simulink subsystem "Orientation"  (R2023b)
settings: Solver=VariableStepAuto  StartTime=0.0  StopTime=10.0  RelTol=1e-3
undefined symbols (not defined in the file or in its folder): DiscIntNeverNeededParam, J, w_wheel1, w_wheel2, w_wheel3
libraries: aerolibutil x3, matrix_library x2, sharedtransform x1, dspmtrx3 x1
settings Model: Creator=andrea  LastModifiedBy=andrea

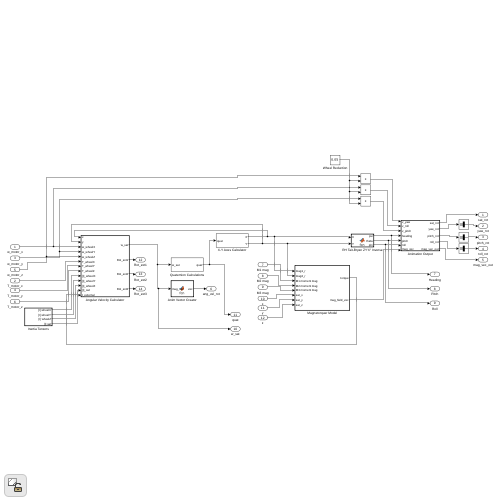
[thumbnail: Simulink's stored preview of the top-level diagram]
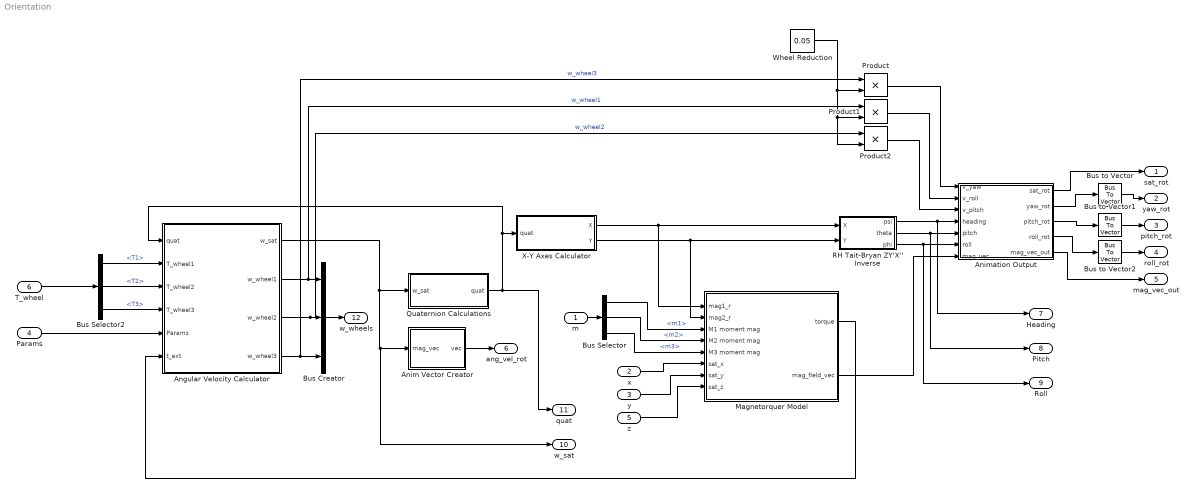
== system Orientation ==
  m : Inport
  x : Inport  Port=2
  y : Inport  Port=3
  Params : Inport  Port=4
  z : Inport  Port=5
  T_wheel : Inport  Port=6
  Angular Velocity Calculator : Subsystem  TreatAsAtomicUnit=on
  Anim Vector Creator : MATLAB Function  TreatAsAtomicUnit=on
  Animation Output : Subsystem  TreatAsAtomicUnit=on
  Bus Creator : BusCreator  Inputs=w_wheel1,w_wheel2,w_wheel3
  Bus Selector : BusSelector  OutputSignals=m1,m2,m3
  Bus Selector2 : BusSelector  OutputSignals=T1,T2,T3
  Bus to Vector : BusToVector
  Bus to Vector1 : BusToVector
  Bus to Vector2 : BusToVector
  Magnetorquer Model : Subsystem  TreatAsAtomicUnit=on
  Product : Product
  Product1 : Product
  Product2 : Product
  Quaternion Calculations : Subsystem
  RH Tait-Bryan ZY'X'' Inverse : MATLAB Function  TreatAsAtomicUnit=on
  Wheel Reduction : Constant  Value=0.05
  X-Y Axes Calculator : Subsystem
  sat_rot : Outport
  yaw_rot : Outport  Port=2
  pitch_rot : Outport  Port=3
  roll_rot : Outport  Port=4
  mag_vec_out : Outport  Port=5
  ang_vel_rot : Outport  Port=6
  Heading : Outport  Port=7
  Pitch : Outport  Port=8
  Roll : Outport  Port=9
  w_sat : Outport  Port=10
  quat : Outport  Port=11
  w_wheels : Outport  Port=12
  wires:
  Animation Output/4(roll_rot) -> Bus to Vector2/1
  Animation Output/3(pitch_rot) -> Bus to Vector1/1
  Bus to Vector1/1 -> pitch_rot/1
  x/1 -> Magnetorquer Model/6(sat_x)
  RH Tait-Bryan ZY'X'' Inverse/3(phi) -> Roll/1, Animation Output/6(roll)
  Wheel Reduction/1 -> Product/2, Product1/2, Product2/2
  Animation Output/1(sat_rot) -> sat_rot/1
  Product1/1 -> Animation Output/2(v_roll)
  Quaternion Calculations/1(quat) -> quat/1, X-Y Axes Calculator/1(quat), Angular Velocity Calculator/1(quat)
  Bus Selector/2 -> Magnetorquer Model/4(M2 moment mag)  "<m2>"
  Angular Velocity Calculator/1(w_sat) -> Anim Vector Creator/1(mag_vec), w_sat/1, Quaternion Calculations/1(w_sat)
  y/1 -> Magnetorquer Model/7(sat_y)
  X-Y Axes Calculator/1(X) -> Magnetorquer Model/1(mag1_r), RH Tait-Bryan ZY'X'' Inverse/1(X)
  z/1 -> Magnetorquer Model/8(sat_z)
  Bus Selector/3 -> Magnetorquer Model/5(M3 moment mag)  "<m3>"
  Bus Selector2/1 -> Angular Velocity Calculator/2(T_wheel1)  "<T1>"
  RH Tait-Bryan ZY'X'' Inverse/2(theta) -> Animation Output/5(pitch), Pitch/1
  Animation Output/5(mag_vec_out) -> mag_vec_out/1
  Bus to Vector2/1 -> roll_rot/1
  Product/1 -> Animation Output/1(v_yaw)
  Animation Output/2(yaw_rot) -> Bus to Vector/1
  Anim Vector Creator/1(vec) -> ang_vel_rot/1
  Product2/1 -> Animation Output/3(v_pitch)
  Bus Selector/1 -> Magnetorquer Model/3(M1 moment mag)  "<m1>"
  RH Tait-Bryan ZY'X'' Inverse/1(psi) -> Heading/1, Animation Output/4(heading)
  X-Y Axes Calculator/2(Y) -> Magnetorquer Model/2(mag2_r), RH Tait-Bryan ZY'X'' Inverse/2(Y)
  Bus to Vector/1 -> yaw_rot/1
  Magnetorquer Model/2(mag_field_vec) -> Animation Output/7(mag_vec)
  Angular Velocity Calculator/2(w_wheel1) -> Bus Creator/1, Product1/1  "w_wheel1"
  Angular Velocity Calculator/3(w_wheel2) -> Bus Creator/2, Product2/1  "w_wheel2"
  Angular Velocity Calculator/4(w_wheel3) -> Bus Creator/3, Product/1  "w_wheel3"
  m/1 -> Bus Selector/1
  T_wheel/1 -> Bus Selector2/1
  Bus Creator/1 -> w_wheels/1
  Params/1 -> Angular Velocity Calculator/5(Params)
  Bus Selector2/2 -> Angular Velocity Calculator/3(T_wheel2)  "<T2>"
  Bus Selector2/3 -> Angular Velocity Calculator/4(T_wheel3)  "<T3>"
  Magnetorquer Model/1(torque) -> Angular Velocity Calculator/6(t_ext)

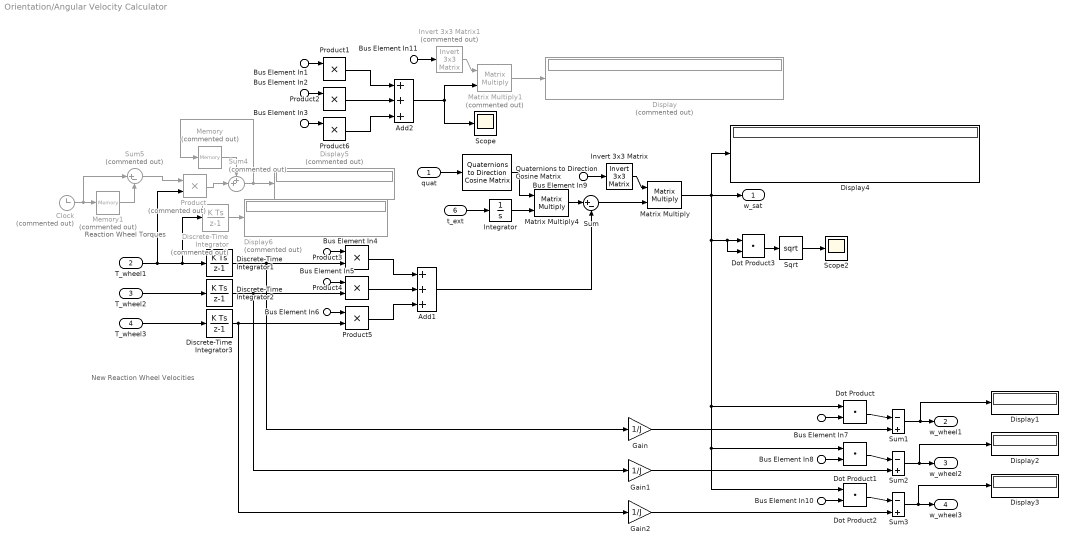
== system Orientation/Angular Velocity Calculator ==
  note: New Reaction Wheel Velocities
  note: Reaction Wheel Torques
  quat : Inport
  T_wheel1 : Inport  Port=2
  T_wheel2 : Inport  Port=3
  T_wheel3 : Inport  Port=4
  Bus Element In9 : Inport  Port=5  PortName=Params  Element=I_sat
  Bus Element In11 : Inport  Port=5  PortName=Params  Element=I_sat
  Bus Element In4 : Inport  Port=5  PortName=Params  Element=a1
  Bus Element In7 : Inport  Port=5  PortName=Params  Element=a1
  Bus Element In1 : Inport  Port=5  PortName=Params  Element=a1
  Bus Element In5 : Inport  Port=5  PortName=Params  Element=a2
  Bus Element In8 : Inport  Port=5  PortName=Params  Element=a2
  Bus Element In2 : Inport  Port=5  PortName=Params  Element=a2
  Bus Element In6 : Inport  Port=5  PortName=Params  Element=a3
  Bus Element In10 : Inport  Port=5  PortName=Params  Element=a3
  Bus Element In3 : Inport  Port=5  PortName=Params  Element=a3
  t_ext : Inport  Port=6
  Add1 : Sum  Inputs=+++
  Add2 : Sum  Inputs=+++
  Clock : Clock  Commented=on
  Discrete-Time Integrator : DiscreteIntegrator  Commented=on  SampleTime=-1  ICPrevOutput=DiscIntNeverNeededParam  ICPrevScaledInput=DiscIntNeverNeededParam
  Discrete-Time Integrator1 : DiscreteIntegrator  SampleTime=-1  ICPrevOutput=DiscIntNeverNeededParam  ICPrevScaledInput=DiscIntNeverNeededParam
  Discrete-Time Integrator2 : DiscreteIntegrator  SampleTime=-1  ICPrevOutput=DiscIntNeverNeededParam  ICPrevScaledInput=DiscIntNeverNeededParam
  Discrete-Time Integrator3 : DiscreteIntegrator  SampleTime=-1  ICPrevOutput=DiscIntNeverNeededParam  ICPrevScaledInput=DiscIntNeverNeededParam
  Display : Display  Commented=on
  Display{1..4} (4 alike) : Display
  Display5 : Display  Commented=on
  Display6 : Display  Commented=on
  Dot Product{,1..3} (4 alike) : DotProduct  OutDataTypeStr=Inherit: Inherit via internal rule
  Gain : Gain  Gain=1/J
  Gain1 : Gain  Gain=1/J
  Gain2 : Gain  Gain=1/J
  Integrator : Integrator
  Invert 3x3 Matrix : aerolibutil/Invert  3x3 Matrix
  Invert 3x3 Matrix1 : aerolibutil/Invert  3x3 Matrix  Commented=on
  Matrix Multiply : Product  Multiplication=Matrix(*)
  Matrix Multiply1 : Product  Commented=on  Multiplication=Matrix(*)
  Matrix Multiply4 : Product  Multiplication=Matrix(*)
  Memory : Memory  Commented=on
  Memory1 : Memory  Commented=on
  Product : Product  Commented=on
  Product{1..6} (6 alike) : Product
  Quaternions to Direction Cosine Matrix : sharedtransform/Quaternions to  Direction Cosine Matrix  aMode=aMode
      settings: LibrarySourceBlock=|
      | aerolibtransform2/Quaternions to
      | Direction Cosine Matrix
  Scope : Scope
  Scope2 : Scope
  Sqrt : Sqrt
  Sum : Sum  Inputs=|+-
  Sum1 : Sum  Inputs=-|+
  Sum2 : Sum  Inputs=-|+
  Sum3 : Sum  Inputs=-|+
  Sum4 : Sum  Commented=on  Inputs=++|
  Sum5 : Sum  Commented=on  Inputs=|+-
  w_sat : Outport
  w_wheel1 : Outport  Port=2
  w_wheel2 : Outport  Port=3
  w_wheel3 : Outport  Port=4
  wires:
  Discrete-Time Integrator/1 -> Display6/1
  T_wheel1/1 -> Discrete-Time Integrator/1, Discrete-Time Integrator1/1, Product/2
  Product/1 -> Sum4/2
  Sum5/1 -> Product/1
  Memory1/1 -> Sum5/2
  Clock/1 -> Memory1/1, Sum5/1
  Sum4/1 -> Memory/1, Display5/1
  Memory/1 -> Sum4/1
  Sqrt/1 -> Scope2/1
  Dot Product3/1 -> Sqrt/1
  Matrix Multiply1/1 -> Display/1
  Add2/1 -> Matrix Multiply1/2, Scope/1
  Bus Element In11/1 -> Invert 3x3 Matrix1/1
  Invert 3x3 Matrix1/1 -> Matrix Multiply1/1
  Bus Element In3/1 -> Product6/1
  Product2/1 -> Add2/2
  Bus Element In2/1 -> Product2/1
  Product6/1 -> Add2/3
  Bus Element In1/1 -> Product1/1
  Product1/1 -> Add2/1
  Matrix Multiply/1 -> Dot Product3/1, Dot Product3/2, Dot Product1/1, Dot Product2/1, Dot Product/1, w_sat/1, Display4/1
  Discrete-Time Integrator3/1 -> Product5/2, Gain2/1
  Discrete-Time Integrator2/1 -> Product4/2, Gain1/1
  Discrete-Time Integrator1/1 -> Product3/2, Gain/1
  Invert 3x3 Matrix/1 -> Matrix Multiply/1
  Sum/1 -> Matrix Multiply/2
  Bus Element In9/1 -> Invert 3x3 Matrix/1
  Matrix Multiply4/1 -> Sum/1
  Integrator/1 -> Matrix Multiply4/2
  Quaternions to Direction Cosine Matrix/1 -> Matrix Multiply4/1
  Add1/1 -> Sum/2
  Gain2/1 -> Sum3/2
  Gain1/1 -> Sum2/2
  Gain/1 -> Sum1/2
  T_wheel3/1 -> Discrete-Time Integrator3/1
  T_wheel2/1 -> Discrete-Time Integrator2/1
  t_ext/1 -> Integrator/1
  quat/1 -> Quaternions to Direction Cosine Matrix/1
  Sum3/1 -> Display3/1, w_wheel3/1
  Sum2/1 -> w_wheel2/1, Display2/1
  Sum1/1 -> w_wheel1/1, Display1/1
  Dot Product2/1 -> Sum3/1
  Dot Product1/1 -> Sum2/1
  Dot Product/1 -> Sum1/1
  Bus Element In10/1 -> Dot Product2/2
  Bus Element In8/1 -> Dot Product1/2
  Bus Element In7/1 -> Dot Product/2
  Bus Element In4/1 -> Product3/1
  Bus Element In5/1 -> Product4/1
  Bus Element In6/1 -> Product5/1
  Product5/1 -> Add1/3
  Product3/1 -> Add1/1
  Product4/1 -> Add1/2

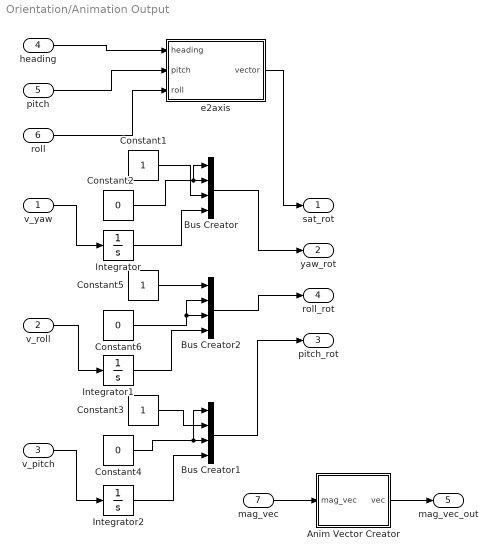
== system Orientation/Animation Output ==
  v_yaw : Inport
  v_roll : Inport  Port=2
  v_pitch : Inport  Port=3
  heading : Inport  Port=4
  pitch : Inport  Port=5
  roll : Inport  Port=6
  mag_vec : Inport  Port=7
  Anim Vector Creator : MATLAB Function  TreatAsAtomicUnit=on
  Bus Creator : BusCreator  Inputs=4
  Bus Creator1 : BusCreator  Inputs=4
  Bus Creator2 : BusCreator  Inputs=4
  Constant1 : Constant
  Constant2 : Constant  Value=0
  Constant3 : Constant
  Constant4 : Constant  Value=0
  Constant5 : Constant
  Constant6 : Constant  Value=0
  Integrator : Integrator
  Integrator1 : Integrator
  Integrator2 : Integrator
  e2axis : MATLAB Function  TreatAsAtomicUnit=on
  sat_rot : Outport
  yaw_rot : Outport  Port=2
  pitch_rot : Outport  Port=3
  roll_rot : Outport  Port=4
  mag_vec_out : Outport  Port=5
  wires:
  Anim Vector Creator/1(vec) -> mag_vec_out/1
  mag_vec/1 -> Anim Vector Creator/1(mag_vec)
  Integrator2/1 -> Bus Creator1/4
  Integrator1/1 -> Bus Creator2/4
  Integrator/1 -> Bus Creator/4
  Bus Creator1/1 -> pitch_rot/1
  Bus Creator2/1 -> roll_rot/1
  Bus Creator/1 -> yaw_rot/1
  v_pitch/1 -> Integrator2/1
  v_roll/1 -> Integrator1/1
  v_yaw/1 -> Integrator/1
  e2axis/1(vector) -> sat_rot/1
  roll/1 -> e2axis/3(roll)
  pitch/1 -> e2axis/2(pitch)
  heading/1 -> e2axis/1(heading)
  Constant4/1 -> Bus Creator1/3, Bus Creator1/1
  Constant2/1 -> Bus Creator/2, Bus Creator/1
  Constant3/1 -> Bus Creator1/2
  Constant1/1 -> Bus Creator/3
  Constant5/1 -> Bus Creator2/1
  Constant6/1 -> Bus Creator2/3, Bus Creator2/2

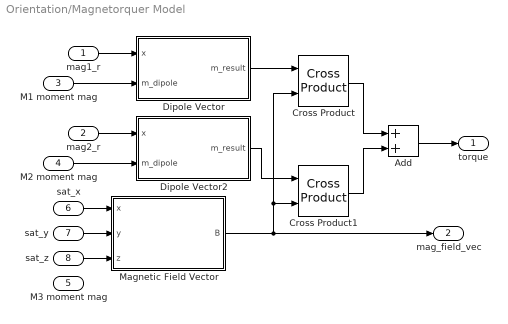
== system Orientation/Magnetorquer Model ==
  mag1_r : Inport
  mag2_r : Inport  Port=2
  M1 moment mag : Inport  Port=3
  M2 moment mag : Inport  Port=4
  M3 moment mag : Inport  Port=5
  sat_x : Inport  Port=6
  sat_y : Inport  Port=7
  sat_z : Inport  Port=8
  Add : Sum
  Cross Product : matrix_library/Cross Product
  Cross Product1 : matrix_library/Cross Product
  Dipole Vector : MATLAB Function  TreatAsAtomicUnit=on
  Dipole Vector2 : MATLAB Function  TreatAsAtomicUnit=on
  Magnetic Field Vector : MATLAB Function  TreatAsAtomicUnit=on
  torque : Outport
  mag_field_vec : Outport  Port=2
  wires:
  mag1_r/1 -> Dipole Vector/1(x)
  mag2_r/1 -> Dipole Vector2/1(x)
  Add/1 -> torque/1
  Dipole Vector/1(m_result) -> Cross Product/1
  M2 moment mag/1 -> Dipole Vector2/2(m_dipole)
  Magnetic Field Vector/1(B) -> Cross Product1/2, Cross Product/2, mag_field_vec/1
  sat_y/1 -> Magnetic Field Vector/2(y)
  sat_z/1 -> Magnetic Field Vector/3(z)
  sat_x/1 -> Magnetic Field Vector/1(x)
  Dipole Vector2/1(m_result) -> Cross Product1/1
  Cross Product/1 -> Add/1
  M1 moment mag/1 -> Dipole Vector/2(m_dipole)
  Cross Product1/1 -> Add/2

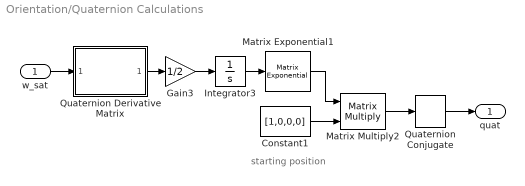
== system Orientation/Quaternion Calculations ==
  note: starting position
  w_sat : Inport
  Constant1 : Constant  Value=[1,0,0,0]
  Gain3 : Gain  Gain=1/2
  Integrator3 : Integrator  InitialCondition=[[0,0,0,0];[0,0,0,0];[0,0,0,0];[0,0,0,0]]
  Matrix Exponential1 : dspmtrx3/Matrix Exponential
  Matrix Multiply2 : Product  Multiplication=Matrix(*)
  Quaternion Conjugate : aerolibutil/Quaternion Conjugate
  Quaternion Derivative Matrix : MATLAB Function  TreatAsAtomicUnit=on
  quat : Outport
  wires:
  Quaternion Conjugate/1 -> quat/1
  w_sat/1 -> Quaternion Derivative Matrix/1(omega)
  Matrix Multiply2/1 -> Quaternion Conjugate/1
  Integrator3/1 -> Matrix Exponential1/1
  Constant1/1 -> Matrix Multiply2/2
  Matrix Exponential1/1 -> Matrix Multiply2/1
  Gain3/1 -> Integrator3/1
  Quaternion Derivative Matrix/1(Omega) -> Gain3/1

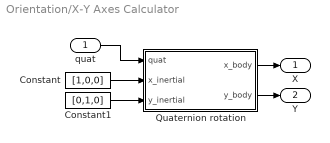
== system Orientation/X-Y Axes Calculator ==
  quat : Inport
  Constant : Constant  Value=[1,0,0]
  Constant1 : Constant  Value=[0,1,0]
  Quaternion rotation : MATLAB Function  TreatAsAtomicUnit=on
  X : Outport
  Y : Outport  Port=2
  wires:
  Quaternion rotation/2(y_body) -> Y/1
  Quaternion rotation/1(x_body) -> X/1
  Constant1/1 -> Quaternion rotation/3(y_inertial)
  Constant/1 -> Quaternion rotation/2(x_inertial)
  quat/1 -> Quaternion rotation/1(quat)

== matlab function Orientation/Animation Output/Anim Vector Creator ==
  data: mag_vec input; vec output
function vec = fcn(mag_vec)

cos_theta = mag_vec(3) / sqrt(mag_vec(1)^2+mag_vec(2)^2+mag_vec(3)^2);
theta = acos(cos_theta);
vec = [-mag_vec(2); mag_vec(1); 0; theta];

== matlab function Orientation/Animation Output/e2axis ==
  data: heading input; pitch input; roll input; vector output

function vector = e2axis(heading, pitch, roll)

eul = [heading -pitch roll];
coder.extrinsic('eul2rotm');
coder.extrinsic('rotm2axang');
rotm = eul2rotm(eul,'ZYX');
v = rotm2axang(rotm);
vector = [0;0;0;0];
vector(1) = v(1);
vector(2) = v(2);
vector(3) = v(3);
vector(4) = v(4);

end

== matlab function Orientation/Magnetorquer Model/Dipole Vector ==
  data: x input; m_result output; m_dipole input
function m_result  = fcn(x,m_dipole)

m_result = [0;0;0];
mag = sqrt(x(1)^2 + x(2)^2 + x(3)^2);
m_result(1) = m_dipole * (x(1) / mag);
m_result(2) = m_dipole * (x(2) / mag);
m_result(3) = m_dipole * (x(3) / mag);

== matlab function Orientation/Magnetorquer Model/Dipole Vector2 ==
  data: x input; m_result output; m_dipole input
function m_result  = fcn(x,m_dipole)

m_result = [0;0;0];
mag = sqrt(x(1)^2 + x(2)^2 + x(3)^2);
m_result(1) = m_dipole * (x(1) / mag);
m_result(2) = m_dipole * (x(2) / mag);
m_result(3) = m_dipole * (x(3) / mag);

== matlab function Orientation/Magnetorquer Model/Magnetic Field Vector ==
  data: x input; B output; y input; z input
function B  = fcn(x,y,z)

B = [0;0;0];
q1 = 150; % bottom charge
q2 = 180; % top charge
r_earth = 6.3781e6;
inset = 2/3;
d_t = x^2 + y^2 + (z - r_earth * inset)^2; % distance squared from top charge to point
d_b = x^2 + y^2 + (z + r_earth * inset)^2; % distance squared from bottom charge to point

B(1) = (x) * (q1 / d_b - q2 / d_t);
B(2) = (y) * (q1 / d_b - q2 / d_t);
B(3) = (q1 / d_b) * (z + r_earth * inset) - (q1 / d_t) * (z - r_earth * inset);

== matlab function Orientation/Quaternion Calculations/Quaternion Derivative Matrix ==
  data: omega input; Omega output
function Omega = fcn(omega)

omega_cell = num2cell(omega);
[omega_x, omega_y, omega_z] = omega_cell{:};

%omega_x = omega(1);
%omega_y = omega(2);
%omega_z = omega(3);

Omega = [[0,            -omega_x,   -omega_y,   -omega_z];
         [omega_x,      0,          -omega_z,    omega_y];
         [omega_y,      omega_z,    0,          -omega_x];
         [omega_z,      -omega_y,   omega_x,    0       ]];

== matlab function Orientation/X-Y Axes Calculator/Quaternion rotation ==
  data: quat input; x_body output; x_inertial input; y_inertial input; y_body output
function [x_body, y_body] = fcn(quat, x_inertial, y_inertial)

x_body = [0,0,0];
y_body = [0,0,0];

%disp("Quaternion:");
%disp(reshape(quat,1,4));
%fprintf(quat);
coder.extrinsic("quat2dcm");
dcm = quat2dcm(reshape(quat,1,4));

x_body = reshape(dcm * x_inertial,1,3);
y_body = reshape(dcm * y_inertial,1,3);


% z_body = x_body x y_body

== matlab function Orientation/Anim Vector Creator ==
  data: mag_vec input; vec output
function vec = fcn(mag_vec)

cos_theta = mag_vec(3) / sqrt(mag_vec(1)^2+mag_vec(2)^2+mag_vec(3)^2);
theta = acos(cos_theta);
vec = [-mag_vec(2); mag_vec(1); 0; theta];

== matlab function Orientation/RH Tait-Bryan ZY'X'' Inverse ==
  data: X input; psi output; theta output; phi output; Y input
function [psi, theta, phi] = fcn(X, Y)

% psi = heading
% theta = pitch
% phi = bank

%eulZYX = [0,0,0];
%coder.extrinsic("quat2eul");
%eulZYX = quat2eul(reshape(quat,1,4));

%psi = eulZYX(1);
%theta = eulZYX(2);
%phi = eulZYX(3);

psi = atan2(X(2),X(1));
theta = atan2(X(3),sqrt(X(2)^2 + X(1)^2));
if(-Y(1) * sin(psi) + Y(2) * cos(psi) > 1)
    n = 1;
elseif(-Y(1) * sin(psi) + Y(2) * cos(psi) < -1)
    n = -1;
else
    n = -Y(1) * sin(psi) + Y(2) * cos(psi);
end
if(Y(3) > 0)
    phi = acos(n);
else
    phi = -acos(n);
end
